simulink model "Matlab_BLCD_commutation_Logic11"  (R2018a)
settings: Solver=VariableStepAuto  StartTime=0.0  StopTime=3  RelTol=1e-3
undefined symbols (not defined in the file or in its folder): Down, Up
libraries: powerlib x9, peBldcCommutationLogic x1, simulink x1, pePwmGenerator x1
settings Model: Creator=User  LastModifiedBy=DELL
settings SolverCC: ZeroCrossAlgorithm=Adaptive
settings DebuggingCC: MaxConsecutiveZCsMsg=none

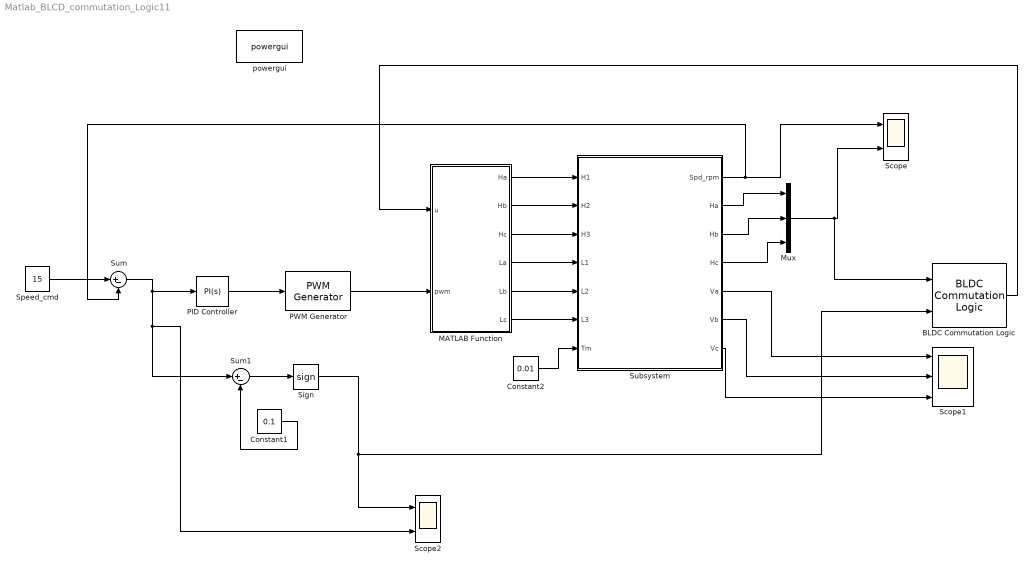
== system Matlab_BLCD_commutation_Logic11 ==
  BLDC Commutation Logic : peBldcCommutationLogic/BLDC Commutation Logic  Ts=-1
  Constant1 : Constant  Value=0.1
  Constant2 : Constant  Value=0.01
  MATLAB Function : MATLAB Function  TreatAsAtomicUnit=on
  Mux : Mux  Inputs=3
  PID Controller : simulink/Continuous/PID Controller  Controller=PI  TimeDomain=Continuous-time  SampleTime=-1  IntegratorMethod=Forward Euler  FilterMethod=Forward Euler  Form=Parallel  UseFilter=on  ControllerParametersSource=internal  P=0.1  I=1  D=0  N=100  InitialConditionSource=internal  InitialConditionForIntegrator=0  InitialConditionForFilter=0  ExternalReset=none  LimitOutput=off  UpperSaturationLimit=inf  LowerSaturationLimit=-inf  LinearizeAsGain=on  AntiWindupMode=none  Kb=1  TrackingMode=off  Kt=1  PParamMin=[]  PParamMax=[]  IParamMin=[]  IParamMax=[]  DParamMin=[]  DParamMax=[]  NParamMin=[]  NParamMax=[]  KbParamMin=[]  KbParamMax=[]  KtParamMin=[]  KtParamMax=[]  POutMin=[]  POutMax=[]  IOutMin=[]  IOutMax=[]  DOutMin=[]  DOutMax=[]  NOutMin=[]  NOutMax=[]  KbOutMin=[]  KbOutMax=[]  KtOutMin=[]  KtOutMax=[]  IntegratorOutMin=[]  IntegratorOutMax=[]  FilterOutMin=[]  FilterOutMax=[]  SumOutMin=[]  SumOutMax=[]  SumI1OutMin=[]  SumI1OutMax=[]  SumI2OutMin=[]  SumI2OutMax=[]  SumI3OutMin=[]  SumI3OutMax=[]  SumDOutMin=[]  SumDOutMax=[]  SaturationOutMin=[]  SaturationOutMax=[]  IntegratorContinuousStateAttributes=''  IntegratorStateMustResolveToSignalObject=off  IntegratorRTWStateStorageClass=Auto  FilterContinuousStateAttributes=''  FilterStateMustResolveToSignalObject=off  FilterRTWStateStorageClass=Auto  DifferentiatorICPrevScaledInput=0  DifferentiatorOutMin=[]  DifferentiatorOutMax=[]  FilterDiffOutCoefMin=[]  FilterDiffOutCoefMax=[]  SumDenOutMin=[]  SumDenOutMax=[]  SumNumOutMin=[]  SumNumOutMax=[]  ReciprocalOutMin=[]  ReciprocalOutMax=[]  DivideOutMin=[]  DivideOutMax=[]  TunerSelectOption=Transfer Function Based (PID Tuner App)
  PWM Generator : pePwmGenerator/PWM Generator  CarrCount=Up-Down  Tper=0.001  Ts=5e-5
  Scope : Scope  NumInputPorts=2
  Scope1 : Scope  NumInputPorts=3
  Scope2 : Scope  NumInputPorts=2
  Sign : Signum
  Speed_cmd : Constant  Value=15
  Subsystem : Subsystem
  Sum : Sum  Inputs=|+-
  Sum1 : Sum  Inputs=|+-
  powergui : powerlib/powergui  Priority=1  SimulationMode=Continuous  SampleTime=50e-6  frequency=60  Iterations=50  frequencyindice=0  Pbase=100e6  ErrMax=1e-4  UnitsV=kV  UnitsW=MW  buscounter=0  FunctionMessages=off  echomessages=off  EnableUseOfTLC=off  CurrentSourceSwitches=off  DisableSnubberDevices=off  DisableRonSwitches=off  DisableVfSwitches=off  DisplayEquations=off  SolverType=Tustin/Backward Euler (TBE)  Interpol=off  ExternalGateDelay=off  methode=off  Ts=100  x0status=blocks  SPID=on  SwTol=0  HookPort=off  RestoreLinks=warning  ResistiveCurrentMeasurement=off  Frange=[0:2:500]  Ylog=off  Xlog=on  ShowGrid=off  save=off  variable=ZData  structure=0  ZoomFFT=off  StartTime=0.0  cycles=1  DisplayStyle=1  fundamental=60  FreqAxis=off  MaxFrequency=1000  frequencyindicesteady=1  RmsSteady=1  display=off
  wires:
  Subsystem/5(Va) -> Scope1/1
  Subsystem/4(Hc) -> Mux/3
  MATLAB Function/5(Lb) -> Subsystem/5(L2)
  Subsystem/7(Vc) -> Scope1/3
  Constant1/1 -> Sum1/2
  Subsystem/6(Vb) -> Scope1/2
  MATLAB Function/1(Ha) -> Subsystem/1(H1)
  MATLAB Function/6(Lc) -> Subsystem/6(L3)
  MATLAB Function/4(La) -> Subsystem/4(L1)
  Subsystem/2(Ha) -> Mux/1
  Constant2/1 -> Subsystem/7(Tm)
  Sum1/1 -> Sign/1
  Mux/1 -> BLDC Commutation Logic/1, Scope/2
  Sign/1 -> Scope2/1, BLDC Commutation Logic/2
  MATLAB Function/2(Hb) -> Subsystem/2(H2)
  BLDC Commutation Logic/1 -> MATLAB Function/1(u)
  Subsystem/3(Hb) -> Mux/2
  Speed_cmd/1 -> Sum/1
  Subsystem/1(Spd_rpm) -> Sum/2, Scope/1
  Sum/1 -> PID Controller/1, Scope2/2, Sum1/1
  PID Controller/1 -> PWM Generator/1
  PWM Generator/1 -> MATLAB Function/2(pwm)
  MATLAB Function/3(Hc) -> Subsystem/3(H3)

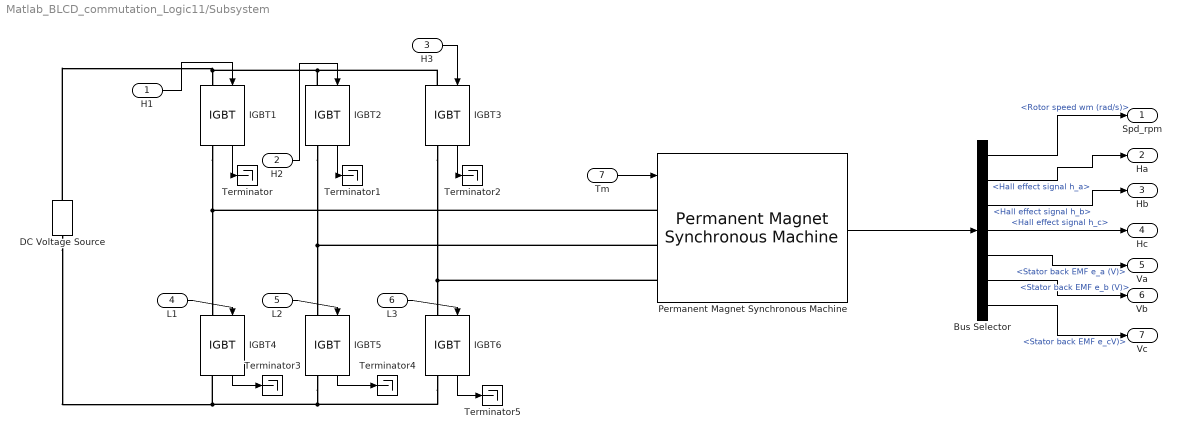
== system Matlab_BLCD_commutation_Logic11/Subsystem ==
  H1 : Inport
  H2 : Inport  Port=2
  H3 : Inport  Port=3
  L1 : Inport  Port=4
  L2 : Inport  Port=5
  L3 : Inport  Port=6
  Tm : Inport  Port=7
  Bus Selector : BusSelector  OutputSignals=Rotor speed wm (rad/s),Hall effect signal h_a,Hall effect signal h_b,Hall effect signal h_c,Stator back EMF e_a (V),Stator back EMF e_b (V),Stator back EMF e_cV)
  DC Voltage Source : powerlib/Electrical Sources/DC Voltage Source  Amplitude=60  Measurements=None
  IGBT{1..6} (6 alike) : powerlib/Power Electronics/IGBT  Ron=0.001  Lon=0  Vf=1  Tf=1e-6  Tt=2e-6  IC=0  Rs=1e5  Cs=inf  Measurements=on
  Permanent Magnet Synchronous Machine : powerlib/Machines/Permanent Magnet Synchronous Machine  NbPhases=3  FluxDistribution=Trapezoidal  RotorType=Round  MechanicalLoad=Torque Tm  PresetModel=No  ShowDetailedParameters=on  MeasurementBus=off  Resistance=0.0485  Inductance=8.5e-3  dqInductances=[8.5e-3,8.5e-3]  La=0.000395  MachineConstant=Flux linkage established by magnets (V.s)  Flux=0.1194  VoltageCst=100.0283  TorqueCst=0.9552  Flat=120  Mechanical=[0.0027 0.0004924 4 0]  PolePairs=4  InitialConditions=[0,0, 0,0]  InitialConditions5ph=[0 0 0 0 0 0]  TsPowergui=0  TsBlock=-1  RefAngle=90 degrees behind phase A axis (modified Park)
      settings: SourceProductName=Simscape Power Systems
  Terminator{,1..5} (6 alike) : Terminator
  Spd_rpm : Outport
  Ha : Outport  Port=2
  Hb : Outport  Port=3
  Hc : Outport  Port=4
  Va : Outport  Port=5
  Vb : Outport  Port=6
  Vc : Outport  Port=7
  wires:
  L1/1 -> IGBT4/1
  Permanent Magnet Synchronous Machine/1 -> Bus Selector/1
  H1/1 -> IGBT1/1
  H2/1 -> IGBT2/1
  H3/1 -> IGBT3/1
  L2/1 -> IGBT5/1
  L3/1 -> IGBT6/1
  Tm/1 -> Permanent Magnet Synchronous Machine/1
  Bus Selector/1 -> Spd_rpm/1  "<Rotor speed wm (rad/s)>"
  Bus Selector/2 -> Ha/1  "<Hall effect signal h_a>"
  Bus Selector/3 -> Hb/1  "<Hall effect signal h_b>"
  Bus Selector/4 -> Hc/1  "<Hall effect signal h_c>"
  Bus Selector/5 -> Va/1  "<Stator back EMF e_a (V)>"
  Bus Selector/6 -> Vb/1  "<Stator back EMF e_b (V)>"
  Bus Selector/7 -> Vc/1  "<Stator back EMF e_cV)>"
  IGBT1/1 -> Terminator/1
  IGBT2/1 -> Terminator1/1
  IGBT3/1 -> Terminator2/1
  IGBT4/1 -> Terminator3/1
  IGBT5/1 -> Terminator4/1
  IGBT6/1 -> Terminator5/1
  connections:
  IGBT3/LConn1 -- IGBT2/LConn1 -- DC Voltage Source/RConn1 -- IGBT1/LConn1
  IGBT6/RConn1 -- IGBT5/RConn1 -- DC Voltage Source/LConn1 -- IGBT4/RConn1
  Permanent Magnet Synchronous Machine/LConn3 -- IGBT3/RConn1 -- IGBT6/LConn1
  Permanent Magnet Synchronous Machine/LConn1 -- IGBT1/RConn1 -- IGBT4/LConn1
  Permanent Magnet Synchronous Machine/LConn2 -- IGBT2/RConn1 -- IGBT5/LConn1

== matlab function Matlab_BLCD_commutation_Logic11/MATLAB Function ==
  data: u input; Ha output; pwm input; Hb output; Hc output; La output; Lb output; Lc output
function [Ha,Hb,Hc,La,Lb,Lc] = fcn(u,pwm)

if u(1)==1
    Ha = 1*pwm;
else
    Ha = 0;
end
if u(1)==-1
    La = 1*pwm;
else
    La = 0;
end
if u(2)==1
    Hb = 1*pwm;
else
    Hb = 0;
end
if u(2)==-1
    Lb = 1*pwm;
else
    Lb = 0; 
end  
if u(3)==1
    Hc = 1*pwm;
else
    Hc = 0;
end
if u(3)==-1
    Lc = 1*pwm;
else
    Lc = 0; 
end
